simulink model "pulchan_r2"  (R2012b)
(part 2 of 91)

  Logical1/1 -> [master_reset]
  [use_self_pps] -> Mux12/1
  self_pps_validation/1(Out1) -> [use_self_pps]
  [arm] -> self_pps_validation/2(allow_modify)
  Delay10/1 -> self_pps_validation/1(In1), Counter2/1
  Constant23/1 -> sync_ctrl/3(sim_3)
  [btm_eth_up] -> tgbe0_linkup/2(out_ten_gbe_1_linkup)
  [top_eth_up] -> tgbe0_linkup/1(out_ten_gbe_0_linkup)
  tgbe0_linkup/1(sim_out) -> Terminator4/1
  tengbe0/2(led_rx) -> Terminator5/1
  tengbe0/12(rx_overrun) -> Terminator13/1
  tengbe0/11(rx_bad_frame) -> Terminator12/1
  tengbe0/10(rx_end_of_frame) -> Terminator11/1
  tengbe0/9(rx_source_port) -> Terminator9/1
  tengbe0/8(rx_source_ip) -> Terminator8/1
  tengbe0/7(rx_valid) -> Terminator7/1
  tengbe0/6(rx_data) -> Terminator6/1
  tengbe1/12(rx_overrun) -> Terminator16/1
  tengbe1/11(rx_bad_frame) -> Terminator15/1
  tengbe1/10(rx_end_of_frame) -> Terminator14/1
  tengbe1/9(rx_source_port) -> Terminator21/1
  tengbe1/8(rx_source_ip) -> Terminator20/1
  tengbe1/7(rx_valid) -> Terminator19/1
  tengbe1/6(rx_data) -> Terminator18/1
  tengbe1/2(led_rx) -> Terminator17/1
  katadc/15(data_valid) -> Terminator22/1
  Constant5/1 -> dest_ip_top/1(sim_1)
  Constant7/1 -> dest_port_top/1(sim_1)
  Constant9/1 -> dest_ip_btm/1(sim_1)
  Constant11/1 -> dest_port_btm/1(sim_1)
  [use_self_pps] -> Mux5/2
  Inverter/1 -> Logical3/1
  [overflow_led] -> Inverter/1
  [clk_bad] -> Inverter1/1
  Inverter1/1 -> Logical3/2
  [btm_eth_up] -> Logical3/3
  [top_eth_up] -> Logical3/4
  [use_self_pps] -> Inverter2/1
  Inverter2/1 -> Logical3/5
  [tx1of] -> latch8/1(set)
  [tx0of] -> latch7/1(set)
  status_reg_ctrl/1(in_of_reset) -> latch4/2(reset), latch8/2(reset), latch7/2(reset), latch6/2(reset), latch5/2(reset), latch3/2(reset), latch2/2(reset), latch1/2(reset), latch/2(reset)
  Constant12/1 -> status_reg_ctrl/1(sim_1)
  Delay/1 -> [buffer_sync_top]
  Delay13/1 -> [frame_count]
  Delay14/1 -> [buffer_dv_top]
  Delay15/1 -> [buffer_data_top]
  Delay16/1 -> [buffer_sync_btm]
  Delay17/1 -> [buffer_dv_btm]
  Delay18/1 -> [buffer_data_btm]
  Delay19/1 -> [heap_size]
  Delay22/1 -> Delay15/1
  Delay21/1 -> Delay14/1
  Delay26/1 -> Delay19/1
  Delay23/1 -> Delay16/1
  Delay20/1 -> Delay/1
  Delay25/1 -> Delay18/1
  Delay24/1 -> Delay17/1
  Delay27/1 -> [band_select]
  Delay28/1 -> tengbe0/2(tx_data)
  Delay29/1 -> tengbe0/3(tx_valid)
  Delay31/1 -> tengbe1/2(tx_data)
  Delay32/1 -> tengbe1/3(tx_valid)
  accumulation_length/1(in_reg) -> Terminator23/1
  Constant22/1 -> accumulation_length/1(sim_1)
  Constant24/1 -> coarse_channel_select/1(sim_1)
  coarse_channel_select/1(in_reg) -> Delay1/1
  Constant25/1 -> digital_gain/1(sim_1)
  digital_gain/1(in_reg) -> Delay3/1
  Constant26/1 -> coarse_fft_shift_mask/1(sim_1)
  coarse_fft_shift_mask/1(in_reg) -> Delay8/1
  Constant14/1 -> tvg_en/1(sim_1)
  sampling_frequency_mhz/1(sim_reg_out) -> Terminator24/1
  Constant17/1 -> Delay34/1
  Delay34/1 -> sampling_frequency_mhz/1(reg_out)
  coarse_fft_size_nsamp/1(sim_reg_out) -> Terminator25/1
  Constant18/1 -> Delay35/1
  Delay35/1 -> coarse_fft_size_nsamp/1(reg_out)
  fine_fft_size_nsamp/1(sim_reg_out) -> Terminator26/1
  Constant19/1 -> Delay36/1
  Delay36/1 -> fine_fft_size_nsamp/1(reg_out)
  Constant1/1 -> adc0_en/1(sim_1)
  Constant4/1 -> adc0_atten/1(sim_1)
  Constant2/1 -> adc1_en/1(sim_1)
  Constant3/1 -> adc1_atten/1(sim_1)
  noise_diode_en/1(in_reg) -> Terminator28/1
  Constant28/1 -> noise_diode_en/1(sim_1)
  noise_diode_duty_cycle_en/1(in_reg) -> Terminator29/1
  Constant29/1 -> noise_diode_duty_cycle_en/1(sim_1)
  noise_diode_on_length/1(in_reg) -> Terminator30/1
  Constant30/1 -> noise_diode_on_length/1(sim_1)
  noise_diode_off_length/1(in_reg) -> Terminator38/1
  Constant32/1 -> noise_diode_off_length/1(sim_1)
  Delay30/1 -> tengbe0/6(tx_end_of_frame)
  Delay33/1 -> tengbe1/6(tx_end_of_frame)
  Gateway Out1/1 -> Scope/1  "sync_in"
  Gateway Out/1 -> Scope/2  "dv_in"
  Gateway Out2/1 -> Scope/3  "dv_out"
